simulink model "threeDofArm_MCGForm"  (R2019b)
settings: Solver=VariableStepAuto  StartTime=0.0  StopTime=30  RelTol=1e-3
settings Model: Creator=OUDUX  LastModifiedBy=Robot
settings DebuggingCC: UnderSpecifiedDimensionMsg=warning

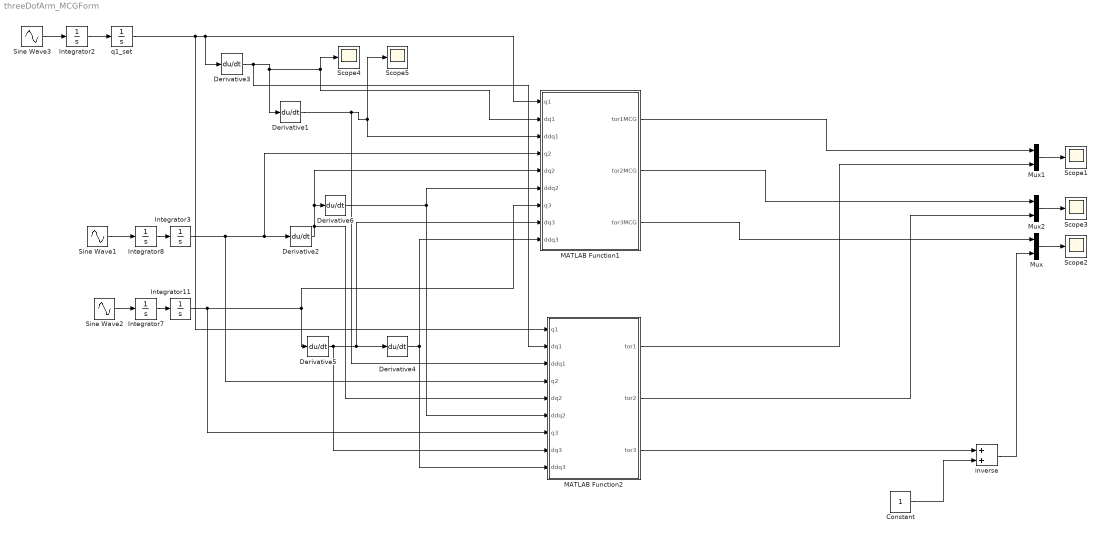
== system threeDofArm_MCGForm ==
  Constant : Constant
  Derivative{1..6} (6 alike) : Derivative
  Integrator{2..3,7..8,11} (5 alike) : Integrator  UpperSaturationLimit=1.57  LowerSaturationLimit=-1.57
  MATLAB Function1 : MATLAB Function  TreatAsAtomicUnit=on
  MATLAB Function2 : MATLAB Function  TreatAsAtomicUnit=on
  Mux : Mux  Inputs=2
  Mux1 : Mux  Inputs=2
  Mux2 : Mux  Inputs=2
  Scope{1..5} (5 alike) : Scope
  Sine Wave1 : Sin  Amplitude=2  SampleTime=0
  Sine Wave2 : Sin  Amplitude=3  SampleTime=0
  Sine Wave3 : Sin  SampleTime=0
  inverse : Sum
  "q1_set " : Integrator  UpperSaturationLimit=1.57  LowerSaturationLimit=-1.57
  wires:
  Mux/1 -> Scope2/1
  Mux2/1 -> Scope3/1
  Mux1/1 -> Scope1/1
  Derivative3/1 -> MATLAB Function2/2(dq1), Scope4/1, MATLAB Function1/2(dq1), Derivative1/1
  Derivative2/1 -> MATLAB Function2/5(dq2), MATLAB Function1/5(dq2), Derivative6/1
  Derivative5/1 -> MATLAB Function2/8(dq3), Derivative4/1, MATLAB Function1/8(dq3)
  Sine Wave3/1 -> Integrator2/1
  Integrator8/1 -> Integrator3/1
  Integrator2/1 -> "q1_set "/1
  Derivative1/1 -> MATLAB Function2/3(ddq1), Scope5/1, MATLAB Function1/3(ddq1)
  Derivative6/1 -> MATLAB Function2/6(ddq2), MATLAB Function1/6(ddq2)
  Derivative4/1 -> MATLAB Function2/9(ddq3), MATLAB Function1/9(ddq3)
  "q1_set "/1 -> MATLAB Function1/1(q1), Derivative3/1, MATLAB Function2/1(q1)
  Integrator3/1 -> MATLAB Function2/4(q2), MATLAB Function1/4(q2), Derivative2/1
  Integrator7/1 -> Integrator11/1
  Integrator11/1 -> MATLAB Function2/7(q3), Derivative5/1, MATLAB Function1/7(q3)
  Sine Wave1/1 -> Integrator8/1
  Sine Wave2/1 -> Integrator7/1
  MATLAB Function1/1(tor1MCG) -> Mux1/1
  MATLAB Function2/1(tor1) -> Mux1/2
  MATLAB Function1/2(tor2MCG) -> Mux2/1
  MATLAB Function2/2(tor2) -> Mux2/2
  MATLAB Function1/3(tor3MCG) -> Mux/1
  inverse/1 -> Mux/2
  MATLAB Function2/3(tor3) -> inverse/1
  Constant/1 -> inverse/2

== matlab function threeDofArm_MCGForm/MATLAB Function1 ==
  data: q1 input; dq1 input; ddq1 input; q2 input; dq2 input; ddq2 input; q3 input; dq3 input; ddq3 input; tor1MCG output; tor2MCG output; tor3MCG output
function [tor1MCG, tor2MCG, tor3MCG] = invDynamicMCG(q1, dq1,ddq1, q2, dq2,ddq2, q3, dq3,ddq3)
    %forwardKinematics
    v0 = [0;0;0;0;0;0];
    Xj1 = Xrotz(q1);
    XT1 = Xtrans([0;0;0]);
    S1 = [0;0;1;0;0;0];
    I1 = mcI(1,[0.5;0;0],[0 0 0;0 0 0;0 0 0.0833]);
    XT2 = Xtrans([1;0;0]);
    Xj2 = Xrotz(q2);
    S2 = [0;0;1;0;0;0];
    I2 = mcI(0.8,[0.4;0;0],[0 0 0;0 0 0;0 0 0.0427]);
    Xj3 = Xrotz(q3);
    XT3 = Xtrans([0.8;0;0]);
    S3 = [0;0;1;0;0;0];
    I3 = mcI(0.6,[0.3;0;0],[0 0 0;0 0 0;0 0 0.0180]); 
    Xup1 =  Xj1 * XT1;
    v1 = Xup1*v0 + S1*dq1;
    Xup2 = Xj2*XT2;
    v2 = Xup2*v1 + S2*dq2;
    Xup3 = Xj3*XT3;
    v3 = Xup3*v2 + S3*dq3;
    %biasAccelerations
    avp0 =[0;0;0;0;0;0];
    avp1 = Xup1*avp0 + crm(v1)*S1*dq1;
    avp2 = Xup2*avp1 + crm(v2)*S2*dq2;
    avp3 = Xup3*avp2 + crm(v3)*S3*dq3;
    %coriolis forces
    fvp1 = I1*avp1 + crf(v1)*I1*v1;
    fvp2 = I2*avp2 + crf(v2)*I2*v2;
    fvp3 = I3*avp3 + crf(v3)*I3*v3;
    C3 = S3'* fvp3;
    fvp2 = fvp2+Xup3'*fvp3;
    C2 = S2'*fvp2;
    fvp1 = fvp1+Xup2'*fvp2;
    C1 = S1'*fvp1;
    %compositeInertias
    IC3 = I3;
    IC2 = I2 + Xup3'*I3*Xup3;
    IC1 = I1 + Xup2'*I2*Xup2;
    %gravityForce
    ag0 = [0;0;0;0;0;0];
    ag1 = Xup1*ag0;
    ag2 = Xup2*ag1;
    ag3 = Xup3*ag2;
    G1 = -S1'*IC1*ag1;
    G2 = -S2'*IC2*ag2;
    G3 = -S3'*IC3*ag3;
    %massMatrix
    F3 = IC3*S3;
    H33 = S3'*F3;
    F3 = Xup3'*F3;
    H32 = F3'*S2;
    H23 = H32';
    F3 = Xup2'*F3;
    H31 = F3'*S1;
    H13 = H31';
    F2 = IC2*S2;
    H22 = S2'*F2;
    F2 = Xup2'*F2;
    H21 = F2'*S1;
    H12 = H21';
    F1 =IC1*S1;
    H11 = S1'*F1;
    Tor = [H11 H12 H13;H21 H22 H23;H31 H32 H33]*[ddq1;ddq2;ddq3];
    tor1MCG = Tor(1,1)+C1+G1;
    tor2MCG = Tor(2,1)+C2+G2;
    tor3MCG = Tor(3,1)+C3+G3;
end

== matlab function threeDofArm_MCGForm/MATLAB Function2 ==
  data: q1 input; dq1 input; ddq1 input; q2 input; dq2 input; ddq2 input; q3 input; dq3 input; ddq3 input; tor1 output; tor2 output; tor3 output
function [tor1, tor2, tor3] = invDynamic(q1, dq1,ddq1, q2, dq2,ddq2, q3, dq3,ddq3)
    a_grav = [0;0;0;0;0;0];
    v0 = [0;0;0;0;0;0];
    Xj1 = Xrotz(q1);
    XT1 = Xtrans([0;0;0]);
    S1 = [0;0;1;0;0;0];
    I1 = mcI(1,[0.5;0;0],[0 0 0;0 0 0;0 0 0.0833]);
    XT2 = Xtrans([1;0;0]);
    Xj2 = Xrotz(q2);
    S2 = [0;0;1;0;0;0];
    I2 = mcI(0.8,[0.4;0;0],[0 0 0;0 0 0;0 0 0.0427]);
    Xj3 = Xrotz(q3);
    XT3 = Xtrans([0.8;0;0]);
    S3 = [0;0;1;0;0;0];
    I3 = mcI(0.6,[0.3;0;0],[0 0 0;0 0 0;0 0 0.0180]); 
    
    Xup1 =  Xj1 * XT1;
    v1 = Xup1*v0 + S1*dq1;
    a1 = Xup1 * -a_grav + S1*ddq1;
    f1 = I1*a1 + crf(v1)*I1*v1;
    Xup2 = Xj2*XT2;
    v2 = Xup2*v1 + S2*dq2;
    a2 = Xup2*a1 + S2*ddq2 + crm(v2)*S2*dq2;
    f2 = I2*a2 + crf(v2)*I2*v2;
    Xup3 = Xj3*XT3;
    v3 = Xup3*v2 + S3*dq3;
    a3 = Xup3*a2 + S3*ddq3 + crm(v3)*S3*dq3;
    f3 = I3*a3 + crf(v3)*I3*v3;
    
    tor3 = S3' * f3;
    f2 = f2 + Xup3'*f3;
    tor2 = S2' *f2;
    f1 = f1 + Xup2' * f2;
    tor1 = S1' * f1;
   
    
    
    
end
